simulink model "Ford_T3T6_ArchCnctnDigrm"  (R2016b)
settings: Solver=FixedStepDiscrete  StartTime=0.0  StopTime=10.0  RelTol=1e-3  EnableMultiTasking=on
libraries: canmsglib x15
(part 9 of 15)

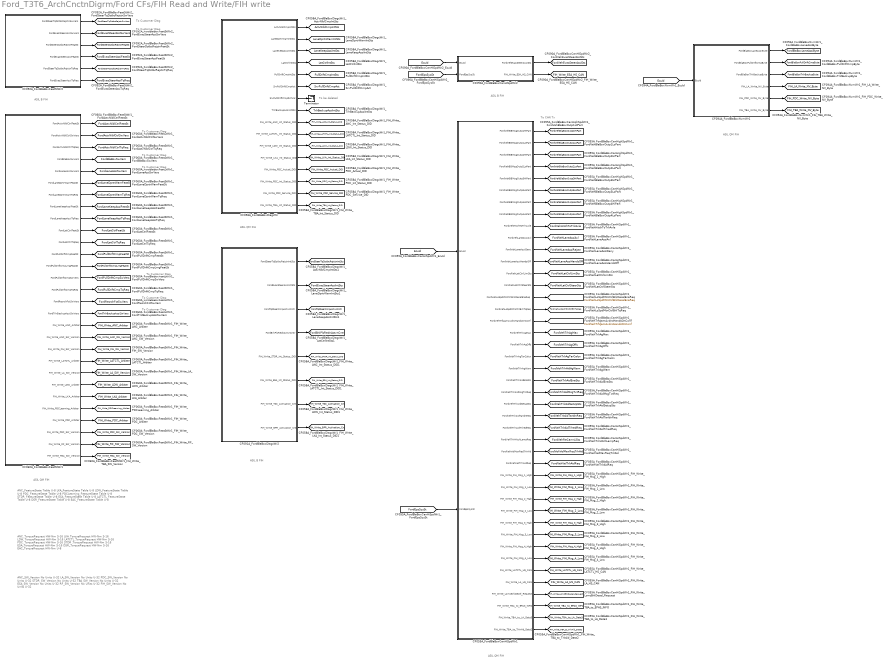
== system Ford_T3T6_ArchCnctnDigrm/Ford CFs/FIH Read and Write/FIH write ==
  note: ASIL QM FIH
  note: ASIL QM FIH
  note: ASIL B FIH
  note: ASIL B FIH
  note: ASIL QM FIH
  note: ASIL QM FIH
  note: ASIL B FIH
  note: To Customer Diag
  note: To be deleted
  note: To CAN Tx
  note: ANC_SW_Version
      | No Units
      | U-32
      |
      | LA_SW_Version
      | No Units
      | U-32
      |
      | PDC_SW_Version
      | No Units
      | U-32
      |
      | STDR_SW_Version
      | No Units
      | U-32
      |
      | TBA_SW_Version
      | No Units
      | U-32
      |
      | ESA_SW_Version
      | No Units
      | U-32
      |
      | RF_SW_Version
      | No Units
      | U-32
      |
      | FIH_SW_Version
      | No Units
      | U-32
  note: ANC_TorqueRequest
      | HW-Nm
      | S-16
      |
      | LKA_TorqueRequest
      | HW-Nm
      | S-16
      |
      | LDW_TorqueRequest
      | HW-Nm
      | S-16
      |
      | LATCTL_TorqueRequest
      | HW-Nm
      | S-16
      |
      | PDC_TorqueRequest
      | HW-Nm
      | S-16
      |
      | STDR_TorqueRequest
      | HW-Nm
      | S-16
      |
      | ESA_TorqueRequest
      | HW-Nm
      | S-16
      |
      | DSR_TorqueRequest
      | HW-Nm
      | S-16
      |
      | EAC_TorqueRequest
      | HW-Nm
      | U-8
  note: ANC_FeatureState
      | Table
      | U-8
      |
      | LKA_FeatureState
      | Table
      | U-8
      |
      | LDW_FeatureState
      | Table
      | U-8
      |
      | PDC_FeatureState
      | Table
      | U-8
      |
      | PDCLearning_FeatureState
      | Table
      | U-8
      |
      | STDR_FeatureState
      | Table
      | U-8
      |
      | ESA_FeatureState
      | Table
      | U-8
      |
      | LATCTL_FeatureState
      | Table
      | U-8
      |
      | DSR_FeatureState
      | Table
      | U-8
      |
      | EAC_FeatureState
      | Table
      | U-8
  note: To Customer Diag
  note: To Customer Diag
  note: To Customer Diag
  note: To Customer Diag
  note: To Customer Diag
  note: To Customer Diag
  note: To Customer Diag
  CF055A_FordBlaBoxCanHiSpdWr1 : Subsystem  Tag=1.0.X  Description=This function passes signals from Ford In House (FIH) features to the CAN bus. This function has no inputs as it is passing through data to the CAN bus from FIH.
      settings: AttributesFormatString=Version: %<Tag>
  CF058A_FordBlaBoxDiagcWr : Subsystem  Tag=1.0.X  Description=The Ford Black Box Diagnostic Write 1 function passes diagnosticinformation from Ford In House (FIH) features to the EPS.
      settings: AttributesFormatString=Version: %<Tag>
  CF060A_FordBlaBoxFeatStWr1 : Subsystem  Tag=1.0.X  Description=The Ford Black Box Feature State Write 1 function allows the Ford In-House (FIH) software,to write information to memory via a specified function call.
      settings: AttributesFormatString=Version: %<Tag>
  CF090A_FordBlaBoxCanHiSpdWr2 : Subsystem  Tag=1.0.X  Description=This function passes signals from Ford In House (FIH) features to the CAN bus. This function has no inputs as it is passing through data to the CAN bus from FIH.
      settings: AttributesFormatString=Version: %<Tag>
  CF091A_FordBlaBoxDiagcWr2 : Subsystem  Tag=1.0.X  Description=The Ford Black Box Diagnostic Write 2 function passes diagnosticinformation from Ford In House (FIH) features to the EPS.
      settings: AttributesFormatString=Version: %<Tag>
  CF092A_FordBlaBoxFeatStWr2 : Subsystem  Tag=1.0.X  Description=The Ford Black Box Feature State Write 2 function allows the Ford In-House (FIH) software, to write information to memory via a specified function call.
      settings: AttributesFormatString=Version: %<Tag>
  CF094A_FordBlaBoxNvmWr1 : Subsystem  Tag=1.0.X  Description=This function allows Ford In House features to read from and write to their specific NVM locations.
      settings: AttributesFormatString=Version: %<Tag>
  Terminator : Terminator
  tag scope: ActvNiblCmpIntSts=global, FIH_LA_Write_NV_Byte=global, FIH_PDC_Write_NV_Byte=global, FIH_TBA_Write_NV_Byte=global, FIH_Write_ANC_Arbiter=global, FIH_Write_ANC_Int_Status_DID=global, FIH_Write_ANC_SW_Version=global, FIH_Write_BPR_Activation_Cnt=global, FIH_Write_ESA_HS_CAN=global, FIH_Write_ESA_Int_Status_DID=global, FIH_Write_FIH_Msg_1_High=global, FIH_Write_FIH_Msg_1_Low=global, FIH_Write_FIH_Msg_2_High=global, FIH_Write_FIH_Msg_2_Low=global, FIH_Write_FIH_Msg_3_High=global, FIH_Write_FIH_Msg_3_Low=global, FIH_Write_FIH_Msg_4_High=global, FIH_Write_FIH_Msg_4_Low=global, FIH_Write_FIH_SW_Version=global, FIH_Write_LATCTL_Arbiter=global, FIH_Write_LATCTL_HS_CAN=global, FIH_Write_LATCTL_Int_Status_DID=global, FIH_Write_LA_HS_CAN=global, FIH_Write_LA_SW_Version=global, FIH_Write_LDW_Arbiter=global, FIH_Write_LDW_Int_Status_DID=global, FIH_Write_LKA_Arbiter=global, FIH_Write_LKA_Int_Status_DID=global, FIH_Write_LsmcBrkDecel_Request=global, FIH_Write_PDCLearning_Arbiter=global, FIH_Write_PDC_Actual_DID=global, FIH_Write_PDC_Arbiter=global, FIH_Write_PDC_Int_Status_DID=global, FIH_Write_PDC_SW_Version=global, FIH_Write_PDC_Service_DID=global, FIH_Write_RF_SW_Version=global, FIH_Write_STDR_Int_Status_DID=global, FIH_Write_TBA_Int_Status_DID=global, FIH_Write_TBA_SW_Version=global, FIH_Write_TBA_to_EPAS_INFO=global, FIH_Write_TBA_to_LA_Data3=global, FIH_Write_TBA_to_TrlrAid_Data2=global, FIH_Write_TSC_Activation_Cnt=global, FordActvNiblCtrlFeatSt=global, FordActvNiblCtrlSwVers=global, FordActvNiblCtrlTqReq=global, FordBlaBoxLaneAssiByte=global, FordBlaBoxPullDriftCmpByte=global, FordBlaBoxSwVers=global, FordBlaBoxTrlrBackupByte=global, FordBrkPlsRednActvnCntr=global, FordEvasSteerAssiFeatSt=global, FordEvasSteerAssiIntSts=global, FordEvasSteerAssiSwVers=global, FordEvasSteerAssiTqReq=global, FordLaneAssiSwVers=global, FordLaneDprtrWarnFeatSt=global, FordLaneDprtrWarnTqReq=global, FordLaneKeepAssiFeatSt=global, FordLaneKeepAssiTqReq=global, FordLatCtrlFeatSt=global, FordLatCtrlTqReq=global, FordPullDriftCmpFeatSt=global, FordPullDriftCmpLrngFeatSt=global, FordPullDriftCmpSwVers=global, FordPullDriftCmpTqReq=global, FordResrchFctSwVers=global, FordSteerDstbcRejctnFeatSt=global, FordSteerTqDstbcRejctnIntSts=global, FordSteerTqDstbcRejctnSwVers=global, FordSteerTqDstbcRejctnTqReq=global, FordTqSteerCmpActvnCntr=global, FordTrlrBackupAssiSwVers=global, FordVehBlaBoxOutp1HiPart=global, FordVehBlaBoxOutp1LoPart=global, FordVehBlaBoxOutp2HiPart=global, FordVehBlaBoxOutp2LoPart=global, FordVehBlaBoxOutp3HiPart=global, FordVehBlaBoxOutp3LoPart=global, FordVehBlaBoxOutp4HiPart=global, FordVehBlaBoxOutp4LoPart=global, FordVehEvasSteerAssiSts=global, FordVehHitchToTrlrAxle=global, FordVehLaneAssiAvl=global, FordVehLaneAssiHandsOff=global, FordVehLaneAssiRejctn=global, FordVehLatCtrlLimSts=global, FordVehLatCtrlSteerSts=global, FordVehLoSpdMtnCtrlBrkDecelEnaReq=global, FordVehLoSpdMtnCtrlBrkTqReq=global, FordVehReCamrLiSts=global, FordVehTrfcJamAvdncHandsOnConf=global, FordVehTrlrAgMax=global, FordVehTrlrAgOffs=global, FordVehTrlrAgTarCalcn=global, FordVehTrlrAidAgWarn=global, FordVehTrlrAidEnaSts=global, FordVehTrlrAidMsgTxtReq=global, FordVehTrlrAidSetUpSts=global, FordVehTrlrAidTarIdnReq=global, FordVehTrlrAidTrlredReq=global, FordVehVelMaxReqTrlrAid=global, FordVehVelTrlrAidReq=global, LaneDprtrWarnIntSts=global, LaneKeepAssiIntSts=global, LatCtrlIntSts=global, PullDriftCmpIntSts=global, SrvPullDriftCmpAct=global, TrlrBackupAssiIntSts=global
  wires:
  CF060A_FordBlaBoxFeatStWr1/1(FordActvNiblCtrlFeatSt) -> [FordActvNiblCtrlFeatSt]
  CF060A_FordBlaBoxFeatStWr1/2(FordActvNiblCtrlSwVers) -> [FordActvNiblCtrlSwVers]
  CF060A_FordBlaBoxFeatStWr1/3(FordActvNiblCtrlTqReq) -> [FordActvNiblCtrlTqReq]
  CF060A_FordBlaBoxFeatStWr1/4(FordBlaBoxSwVers) -> [FordBlaBoxSwVers]
  CF060A_FordBlaBoxFeatStWr1/5(FordLaneAssiSwVers) -> [FordLaneAssiSwVers]
  CF060A_FordBlaBoxFeatStWr1/6(FordLaneDprtrWarnFeatSt) -> [FordLaneDprtrWarnFeatSt]
  CF060A_FordBlaBoxFeatStWr1/7(FordLaneDprtrWarnTqReq) -> [FordLaneDprtrWarnTqReq]
  CF060A_FordBlaBoxFeatStWr1/8(FordLaneKeepAssiFeatSt) -> [FordLaneKeepAssiFeatSt]
  CF060A_FordBlaBoxFeatStWr1/9(FordLaneKeepAssiTqReq) -> [FordLaneKeepAssiTqReq]
  CF060A_FordBlaBoxFeatStWr1/10(FordLatCtrlFeatSt) -> [FordLatCtrlFeatSt]
  CF060A_FordBlaBoxFeatStWr1/11(FordLatCtrlTqReq) -> [FordLatCtrlTqReq]
  CF060A_FordBlaBoxFeatStWr1/12(FordPullDriftCmpFeatSt) -> [FordPullDriftCmpFeatSt]
  CF060A_FordBlaBoxFeatStWr1/13(FordPullDriftCmpLrngFeatSt) -> [FordPullDriftCmpLrngFeatSt]
  CF060A_FordBlaBoxFeatStWr1/14(FordPullDriftCmpSwVers) -> [FordPullDriftCmpSwVers]
  CF060A_FordBlaBoxFeatStWr1/15(FordPullDriftCmpTqReq) -> [FordPullDriftCmpTqReq]
  CF060A_FordBlaBoxFeatStWr1/16(FordResrchFctSwVers) -> [FordResrchFctSwVers]
  CF060A_FordBlaBoxFeatStWr1/17(FordTrlrBackupAssiSwVers) -> [FordTrlrBackupAssiSwVers]
  CF060A_FordBlaBoxFeatStWr1/18(FIH_Write_ANC_Arbiter) -> [FIH_Write_ANC_Arbiter]
  CF060A_FordBlaBoxFeatStWr1/19(FIH_Write_ANC_SW_Version) -> [FIH_Write_ANC_SW_Version]
  CF060A_FordBlaBoxFeatStWr1/20(FIH_Write_FIH_SW_Version) -> [FIH_Write_FIH_SW_Version]
  CF060A_FordBlaBoxFeatStWr1/21(FIH_Write_LATCTL_Arbiter) -> [FIH_Write_LATCTL_Arbiter]
  CF060A_FordBlaBoxFeatStWr1/22(FIH_Write_LA_SW_Version) -> [FIH_Write_LA_SW_Version]
  CF060A_FordBlaBoxFeatStWr1/23(FIH_Write_LDW_Arbiter) -> [FIH_Write_LDW_Arbiter]
  CF060A_FordBlaBoxFeatStWr1/24(FIH_Write_LKA_Arbiter) -> [FIH_Write_LKA_Arbiter]
  CF060A_FordBlaBoxFeatStWr1/25(FIH_Write_PDCLearning_Arbiter) -> [FIH_Write_PDCLearning_Arbiter]
  CF060A_FordBlaBoxFeatStWr1/26(FIH_Write_PDC_Arbiter) -> [FIH_Write_PDC_Arbiter]
  CF060A_FordBlaBoxFeatStWr1/27(FIH_Write_PDC_SW_Version) -> [FIH_Write_PDC_SW_Version]
  CF060A_FordBlaBoxFeatStWr1/28(FIH_Write_RF_SW_Version) -> [FIH_Write_RF_SW_Version]
  CF060A_FordBlaBoxFeatStWr1/29(FIH_Write_TBA_SW_Version) -> [FIH_Write_TBA_SW_Version]
  CF058A_FordBlaBoxDiagcWr/1(ActvNiblCmpIntSts) -> [ActvNiblCmpIntSts]
  CF058A_FordBlaBoxDiagcWr/2(LaneDprtrWarnIntSts) -> [LaneDprtrWarnIntSts]
  CF058A_FordBlaBoxDiagcWr/3(LaneKeepAssiIntSts) -> [LaneKeepAssiIntSts]
  CF058A_FordBlaBoxDiagcWr/4(LatCtrlIntSts) -> [LatCtrlIntSts]
  CF058A_FordBlaBoxDiagcWr/5(PullDriftCmpIntSts) -> [PullDriftCmpIntSts]
  CF058A_FordBlaBoxDiagcWr/6(SrvPullDriftCmpAct) -> [SrvPullDriftCmpAct]
  CF058A_FordBlaBoxDiagcWr/7(SrvPullDriftCmpRstVal) -> Terminator/1
  CF058A_FordBlaBoxDiagcWr/8(TrlrBackupAssiIntSts) -> [TrlrBackupAssiIntSts]
  CF058A_FordBlaBoxDiagcWr/9(FIH_Write_ANC_Int_Status_DID) -> [FIH_Write_ANC_Int_Status_DID]
  CF058A_FordBlaBoxDiagcWr/10(FIH_Write_LATCTL_Int_Status_DID) -> [FIH_Write_LATCTL_Int_Status_DID]
  CF058A_FordBlaBoxDiagcWr/11(FIH_Write_LDW_Int_Status_DID) -> [FIH_Write_LDW_Int_Status_DID]
  CF058A_FordBlaBoxDiagcWr/12(FIH_Write_LKA_Int_Status_DID) -> [FIH_Write_LKA_Int_Status_DID]
  CF058A_FordBlaBoxDiagcWr/13(FIH_Write_PDC_Actual_DID) -> [FIH_Write_PDC_Actual_DID]
  CF058A_FordBlaBoxDiagcWr/14(FIH_Write_PDC_Int_Status_DID) -> [FIH_Write_PDC_Int_Status_DID]
  CF058A_FordBlaBoxDiagcWr/15(FIH_Write_PDC_Service_DID) -> [FIH_Write_PDC_Service_DID]
  CF058A_FordBlaBoxDiagcWr/16(FIH_Write_TBA_Int_Status_DID) -> [FIH_Write_TBA_Int_Status_DID]
  [EcuId] -> CF090A_FordBlaBoxCanHiSpdWr2/1(EcuId)
  [FordEpsSysSt] -> CF090A_FordBlaBoxCanHiSpdWr2/2(FordEpsSysSt)
  CF090A_FordBlaBoxCanHiSpdWr2/1(FordVehEvasSteerAssiSts) -> [FordVehEvasSteerAssiSts]
  CF090A_FordBlaBoxCanHiSpdWr2/2(FIH_Write_ESA_HS_CAN) -> [FIH_Write_ESA_HS_CAN]
  [EcuId] -> CF094A_FordBlaBoxNvmWr1/1(EcuId)
  CF094A_FordBlaBoxNvmWr1/1(FordBlaBoxLaneAssiByte) -> [FordBlaBoxLaneAssiByte]
  CF094A_FordBlaBoxNvmWr1/2(FordBlaBoxPullDriftCmpByte) -> [FordBlaBoxPullDriftCmpByte]
  CF094A_FordBlaBoxNvmWr1/3(FordBlaBoxTrlrBackupByte) -> [FordBlaBoxTrlrBackupByte]
  CF094A_FordBlaBoxNvmWr1/4(FIH_LA_Write_NV_Byte) -> [FIH_LA_Write_NV_Byte]
  CF094A_FordBlaBoxNvmWr1/5(FIH_PDC_Write_NV_Byte) -> [FIH_PDC_Write_NV_Byte]
  CF094A_FordBlaBoxNvmWr1/6(FIH_TBA_Write_NV_Byte) -> [FIH_TBA_Write_NV_Byte]
  CF092A_FordBlaBoxFeatStWr2/1(FordSteerTqDstbcRejctnSwVers) -> [FordSteerTqDstbcRejctnSwVers]
  CF092A_FordBlaBoxFeatStWr2/2(FordEvasSteerAssiSwVers) -> [FordEvasSteerAssiSwVers]
  CF092A_FordBlaBoxFeatStWr2/3(FordSteerDstbcRejctnFeatSt) -> [FordSteerDstbcRejctnFeatSt]
  CF092A_FordBlaBoxFeatStWr2/4(FordEvasSteerAssiFeatSt) -> [FordEvasSteerAssiFeatSt]
  CF092A_FordBlaBoxFeatStWr2/5(FordSteerTqDstbcRejctnTqReq) -> [FordSteerTqDstbcRejctnTqReq]
  CF092A_FordBlaBoxFeatStWr2/6(FordEvasSteerAssiTqReq) -> [FordEvasSteerAssiTqReq]
  [EcuId] -> CF055A_FordBlaBoxCanHiSpdWr1/1(EcuId)
  [FordEpsSysSt] -> CF055A_FordBlaBoxCanHiSpdWr1/2(FordEpsSysSt)
  CF055A_FordBlaBoxCanHiSpdWr1/1(FordVehBBMsgOutp1HiPart) -> [FordVehBlaBoxOutp1HiPart]
  CF055A_FordBlaBoxCanHiSpdWr1/2(FordVehBBMsgOutp1LoPart) -> [FordVehBlaBoxOutp1LoPart]
  CF055A_FordBlaBoxCanHiSpdWr1/3(FordVehBBMsgOutp2HiPart) -> [FordVehBlaBoxOutp2HiPart]
  CF055A_FordBlaBoxCanHiSpdWr1/4(FordVehBBMsgOutp2LoPart) -> [FordVehBlaBoxOutp2LoPart]
  CF055A_FordBlaBoxCanHiSpdWr1/5(FordVehBBMsgOutp3HiPart) -> [FordVehBlaBoxOutp3HiPart]
  CF055A_FordBlaBoxCanHiSpdWr1/6(FordVehBBMsgOutp3LoPart) -> [FordVehBlaBoxOutp3LoPart]
  CF055A_FordBlaBoxCanHiSpdWr1/7(FordVehBBMsgOutp4HiPart) -> [FordVehBlaBoxOutp4HiPart]
  CF055A_FordBlaBoxCanHiSpdWr1/8(FordVehBBMsgOutp4LoPart) -> [FordVehBlaBoxOutp4LoPart]
  CF055A_FordBlaBoxCanHiSpdWr1/9(FordVehHitchToTrlrAxle) -> [FordVehHitchToTrlrAxle]
  CF055A_FordBlaBoxCanHiSpdWr1/10(FordVehLaneAssiAvl) -> [FordVehLaneAssiAvl]
  CF055A_FordBlaBoxCanHiSpdWr1/11(FordVehLaneAssiDeny) -> [FordVehLaneAssiRejctn]
  CF055A_FordBlaBoxCanHiSpdWr1/12(FordVehLaneAssiHandsOff) -> [FordVehLaneAssiHandsOff]
  CF055A_FordBlaBoxCanHiSpdWr1/13(FordVehLatCtrlLimSts) -> [FordVehLatCtrlLimSts]
  CF055A_FordBlaBoxCanHiSpdWr1/14(FordVehLatCtrlSteerSts) -> [FordVehLatCtrlSteerSts]
  CF055A_FordBlaBoxCanHiSpdWr1/15(FordVehLoSpdMtnCtrlBrkDecelEnaReq) -> [FordVehLoSpdMtnCtrlBrkDecelEnaReq]
  CF055A_FordBlaBoxCanHiSpdWr1/16(FordVehLoSpdMtnCtrlBrkTqReq) -> [FordVehLoSpdMtnCtrlBrkTqReq]
  CF055A_FordBlaBoxCanHiSpdWr1/17(FordVehTrfcJamAvdncHandsOnConf) -> [FordVehTrfcJamAvdncHandsOnConf]
  CF055A_FordBlaBoxCanHiSpdWr1/18(FordVehTrlrAgMax) -> [FordVehTrlrAgMax]
  CF055A_FordBlaBoxCanHiSpdWr1/19(FordVehTrlrAgOffs) -> [FordVehTrlrAgOffs]
  CF055A_FordBlaBoxCanHiSpdWr1/20(FordVehTrlrAgTarCalcn) -> [FordVehTrlrAgTarCalcn]
  CF055A_FordBlaBoxCanHiSpdWr1/21(FordVehTrlrAgWarn) -> [FordVehTrlrAidAgWarn]
  CF055A_FordBlaBoxCanHiSpdWr1/22(FordVehTrlrAidEnaSts) -> [FordVehTrlrAidEnaSts]
  CF055A_FordBlaBoxCanHiSpdWr1/23(FordVehTrlrAidMsgTxtReq) -> [FordVehTrlrAidMsgTxtReq]
  CF055A_FordBlaBoxCanHiSpdWr1/24(FordVehTrlrAidSetupSts) -> [FordVehTrlrAidSetUpSts]
  CF055A_FordBlaBoxCanHiSpdWr1/25(FordVehTrlrAidTarIdnReq) -> [FordVehTrlrAidTarIdnReq]
  CF055A_FordBlaBoxCanHiSpdWr1/26(FordVehTrlrAidTrlredReq) -> [FordVehTrlrAidTrlredReq]
  CF055A_FordBlaBoxCanHiSpdWr1/27(FordVehTrlrHitchLampReq) -> [FordVehReCamrLiSts]
  CF055A_FordBlaBoxCanHiSpdWr1/28(FordVehVelMaxReqTrlrAid) -> [FordVehVelMaxReqTrlrAid]
  CF055A_FordBlaBoxCanHiSpdWr1/29(FordVehVelTrlrAidReq) -> [FordVehVelTrlrAidReq]
  CF055A_FordBlaBoxCanHiSpdWr1/30(FIH_Write_FIH_Msg_1_High) -> [FIH_Write_FIH_Msg_1_High]
  CF055A_FordBlaBoxCanHiSpdWr1/31(FIH_Write_FIH_Msg_1_Low) -> [FIH_Write_FIH_Msg_1_Low]
  CF055A_FordBlaBoxCanHiSpdWr1/32(FIH_Write_FIH_Msg_2_High) -> [FIH_Write_FIH_Msg_2_High]
  CF055A_FordBlaBoxCanHiSpdWr1/33(FIH_Write_FIH_Msg_2_Low) -> [FIH_Write_FIH_Msg_2_Low]
  CF055A_FordBlaBoxCanHiSpdWr1/34(FIH_Write_FIH_Msg_3_High) -> [FIH_Write_FIH_Msg_3_High]
  CF055A_FordBlaBoxCanHiSpdWr1/35(FIH_Write_FIH_Msg_3_Low) -> [FIH_Write_FIH_Msg_3_Low]
  CF055A_FordBlaBoxCanHiSpdWr1/36(FIH_Write_FIH_Msg_4_High) -> [FIH_Write_FIH_Msg_4_High]
  CF055A_FordBlaBoxCanHiSpdWr1/37(FIH_Write_FIH_Msg_4_Low) -> [FIH_Write_FIH_Msg_4_Low]
  CF055A_FordBlaBoxCanHiSpdWr1/38(FIH_Write_LATCTL_HS_CAN) -> [FIH_Write_LATCTL_HS_CAN]
  CF055A_FordBlaBoxCanHiSpdWr1/39(FIH_Write_LA_HS_CAN) -> [FIH_Write_LA_HS_CAN]
  CF055A_FordBlaBoxCanHiSpdWr1/40(FIH_Write_LsmcBrkDecel_Request) -> [FIH_Write_LsmcBrkDecel_Request]
  CF055A_FordBlaBoxCanHiSpdWr1/41(FIH_Write_TBA_to_EPAS_INFO) -> [FIH_Write_TBA_to_EPAS_INFO]
  CF055A_FordBlaBoxCanHiSpdWr1/42(FIH_Write_TBA_to_LA_Data3) -> [FIH_Write_TBA_to_LA_Data3]
  CF055A_FordBlaBoxCanHiSpdWr1/43(FIH_Write_TBA_to_TrlrAid_Data2) -> [FIH_Write_TBA_to_TrlrAid_Data2]
  CF091A_FordBlaBoxDiagcWr2/1(FordSteerTqDstbcRejctnIntSts) -> [FordSteerTqDstbcRejctnIntSts]
  CF091A_FordBlaBoxDiagcWr2/2(FordEvasSteerAssiIntSts) -> [FordEvasSteerAssiIntSts]
  CF091A_FordBlaBoxDiagcWr2/3(FordTqSteerCmpActvnCntr) -> [FordTqSteerCmpActvnCntr]
  CF091A_FordBlaBoxDiagcWr2/4(FordBrkPlsRednActvnCntr) -> [FordBrkPlsRednActvnCntr]
  CF091A_FordBlaBoxDiagcWr2/5(FIH_Write_STDR_Int_Status_DID) -> [FIH_Write_STDR_Int_Status_DID]
  CF091A_FordBlaBoxDiagcWr2/6(FIH_Write_ESA_Int_Status_DID) -> [FIH_Write_ESA_Int_Status_DID]
  CF091A_FordBlaBoxDiagcWr2/7(FIH_Write_TSC_Activation_Cnt) -> [FIH_Write_TSC_Activation_Cnt]
  CF091A_FordBlaBoxDiagcWr2/8(FIH_Write_BPR_Activation_Cnt) -> [FIH_Write_BPR_Activation_Cnt]

== system Ford_T3T6_ArchCnctnDigrm/Ford CFs/Internal CF/CF046A_FordVltgIf ==
  BattRtnCurr : Inport
  BattRtnCurrImc : Inport  Port=2
  BattVltg : Inport  Port=3
  FordActvParkAssiEnad : Inport  Port=4
  FordEpsSysSt : Inport  Port=5
  FordEvasSteerAssiEnad : Inport  Port=6
  FordLaneCentrAssiEnad : Inport  Port=7
  FordLaneDprtrWarnEnad : Inport  Port=8
  FordLaneKeepAssiEnad : Inport  Port=9
  FordMaxAsscTq : Inport  Port=10
  FordSysSt : Inport  Port=11
  FordTrfcJamAssiEnad : Inport  Port=12
  FordTrlrBackupAssiEnad : Inport  Port=13
  FordVehElecPwrStrtStopSts : Inport  Port=14
  FordVehElecPwrSts : Inport  Port=15
  FordVehIgnStsQly : Inport  Port=16
  FordVehPwrpkTqSts : Inport  Port=17
  FordVehSpd : Inport  Port=18
  FordVehSpdVld : Inport  Port=19
  GetRefTmr100MicroSec32bit : Inport  Port=20
  GetTiSpan100MicroSec32bit : Inport  Port=21
  SetNtcSts : Inport  Port=22
  FordEpsCurr : Outport
  FordEpsVltg : Outport  Port=2
  FordFeatThdSts : Outport  Port=3
  FordInhbBattVltgDiagc : Outport  Port=4
  FordMaxBattCurr : Outport  Port=5
  FordMinBattVltg : Outport  Port=6
  FordVltgOperRamp : Outport  Port=7
  FordVltgOperScar : Outport  Port=8
  FordVltgOperSt : Outport  Port=9

== system Ford_T3T6_ArchCnctnDigrm/Ford CFs/Internal CF/CF047A_FordStrtStop ==
  CmpdSteerPinionAg : Inport
  CmpdSteerPinionAgQlyFac : Inport  Port=2
  EcuId : Inport  Port=3
  FildVehSpd : Inport  Port=4
  FordBoostCrvInpTq : Inport  Port=5
  FordCanDtcInhb : Inport  Port=6
  FordEpsSysSt : Inport  Port=7
  FordVehElecPwrStrtStopSts : Inport  Port=8
  SteerPinionAgVel : Inport  Port=9
  SteerPinionAgVelVld : Inport  Port=10
  StrtStopDIDSt : Inport  Port=11
  GetRefTmr100MicroSec32bit : Inport  Port=12
  GetSigImcData_logl : Inport  Port=13
  GetSigImcData_u08 : Inport  Port=14
  GetTiSpan100MicroSec32bit : Inport  Port=15
  FordIntPwrReqSt : Outport
  FordIntStrtStopSt : Outport  Port=2
  FordPwrReqSt : Outport  Port=3
  SysOperMotTqCmdSca : Outport  Port=4
  SysOperRampRate : Outport  Port=5

== system Ford_T3T6_ArchCnctnDigrm/Ford CFs/Internal CF/CF048A_DrvrSteerRcmdn ==
  DSRVld : Inport
  DSR_ArbiterCmd : Inport  Port=2
  DSR_Enad : Inport  Port=3
  DrvSte_D_Stat : Inport  Port=4
  DrvSte_Tq_Rq : Inport  Port=5
  EcuId : Inport  Port=6
  RvsGearVld : Inport  Port=7
  VehSpdVld : Inport  Port=8
  GetImcSigData_f32 : Inport  Port=9
  GetImcSigData_logl : Inport  Port=10
  GetImcSigData_u08 : Inport  Port=11
  DSR_FeatSt_PostImc : Outport
  DSR_FeatSt_PreImc : Outport  Port=2
  DSR_TqReq_PostImc : Outport  Port=3
  DSR_TqReq_PreImc : Outport  Port=4
  DrvSteAct_B_Stat_PostImc : Outport  Port=5
  DrvSteAct_B_Stat_PreImc : Outport  Port=6
  DrvSte_Tq_Act : Outport  Port=7

== system Ford_T3T6_ArchCnctnDigrm/Ford CFs/Internal CF/CF050A_FordCanDtcInhb ==
  EcuId : Inport
  FordBattVltgEstimn : Inport  Port=2
  FordEpsSysSt : Inport  Port=3
  FordVehElecPwrSts : Inport  Port=4
  FordVehIgnStsQly : Inport  Port=5
  FordVehLifeCycModQly : Inport  Port=6
  FordVehPwrpkTqSts : Inport  Port=7
  GetRefTmr100MicroSec32bit : Inport  Port=8
  GetSigImcData_logl : Inport  Port=9
  GetSigImcData_u08 : Inport  Port=10
  GetTiSpan100MicroSec32bit : Inport  Port=11
  IoHwAb_GetGpioMcuEna : Inport  Port=12
  OdomMstVal : Inport  Port=13
  FordCanDtcInhb : Outport
  FordEpsLifeCycMod : Outport  Port=2

== system Ford_T3T6_ArchCnctnDigrm/Ford CFs/Internal CF/CF052A_FordSysSt ==
  IoHwAb_GetGpioMcuEna : Inport
  LoaSt : Inport  Port=2
  SysSt : Inport  Port=3
  FordVehPwrpkTqSts : Inport  Port=4
  FordVehSpd : Inport  Port=5
  FordVehSpdVld : Inport  Port=6
  FordVltgOperSt : Inport  Port=7
  GetNtcQlfrSts : Inport  Port=8
  FordEpsFailr : Outport
  FordEpsSysSt : Outport  Port=2
  FordPwrSplyEnaReq : Outport  Port=3
  FordSteerModlSts : Outport  Port=4
  FordEpsEna : Outport  Port=5
  FordSysStReqEna : Outport  Port=6

== system Ford_T3T6_ArchCnctnDigrm/Ford CFs/Internal CF/CF063A_DrvgSteerSel ==
  ActvRtIdx : Inport
  BoostCrvInpTq : Inport  Port=2
  EcuId : Inport  Port=3
  EpsSysSt : Inport  Port=4
  FltMtgtn : Inport  Port=5
  LoaSt : Inport  Port=6
  SelvDrvgModChassis2Req : Inport  Port=7
  SelvDrvgModChassisVld : Inport  Port=8
  SelvDrvgModEnad : Inport  Port=9
  VehSpd : Inport  Port=10
  VehSpdVld : Inport  Port=11
  GetRefTmr100MicroSec32bit : Inport  Port=12
  GetSigImcData_u08 : Inport  Port=13
  GetTiSpan100MicroSec32bit : Inport  Port=14
  RtCalChgReqSts : Outport
  SelvDrvgModSteerModReq : Outport  Port=2
  SelvDrvgModSteerSts : Outport  Port=3
  XcpCalChgReqSts : Outport  Port=4
  RtReqSrv : Outport  Port=5
  XcpReqSrv : Outport  Port=6

== system Ford_T3T6_ArchCnctnDigrm/Ford CFs/Internal CF/CF065A_FordCmdArbn ==
  EcuId : Inport
  FordActvNiblCtrlFeatSt : Inport  Port=2
  FordDrvrSteerRcmdnFeatSt : Inport  Port=3
  FordEvasSteerAssiFeatSt : Inport  Port=4
  FordExtAgCtrlFeatSt : Inport  Port=5
  FordLaneDprtrWarnFeatSt : Inport  Port=6
  FordLaneKeepAssiFeatSt : Inport  Port=7
  FordLatCtrlFeatSt : Inport  Port=8
  FordMaxAssiTq : Inport  Port=9
  FordPullDriftCmpFeatSt : Inport  Port=10
  FordPullDriftCmpLrngFeatSt : Inport  Port=11
  FordSpare1FeatSt : Inport  Port=12
  FordSpare2FeatSt : Inport  Port=13
  FordSpare3FeatSt : Inport  Port=14
  FordSteerDstbcRejctnFeatSt : Inport  Port=15
  FordSteerModlSts : Inport  Port=16
  GetSigImcData_u08 : Inport  Port=17
  FordActvNiblCtrlArbnCmd : Outport
  FordDrvrSteerRcmdnArbnCmd : Outport  Port=2
  FordEvasSteerAssiArbnCmd : Outport  Port=3
  FordExtAgCtrlArbnCmd : Outport  Port=4
  FordLaneDprtrWarnArbnCmd : Outport  Port=5
  FordLaneKeepAssiArbnCmd : Outport  Port=6
  FordLatCtrlArbnCmd : Outport  Port=7
  FordPullDriftCmpArbnCmd : Outport  Port=8
  FordPullDriftCmpLrngArbnCmd : Outport  Port=9
  FordSpare1ArbnCmd : Outport  Port=10
  FordSpare2ArbnCmd : Outport  Port=11
  FordSpare3ArbnCmd : Outport  Port=12
  FordSteerDstbcRejctnArbnCmd : Outport  Port=13

== system Ford_T3T6_ArchCnctnDigrm/Ford CFs/Internal CF/CF066A_FordMotTqCmdOvrlLimr ==
  EcuId : Inport
  FildHwTq : Inport  Port=2
  FildVehSpd : Inport  Port=3
  FordActvNiblCtrlArbnCmd : Inport  Port=4
  FordActvNiblCtrlFctCallSts : Inport  Port=5
  FordActvNiblCtrlTqReq : Inport  Port=6
  FordLaneDprtrWarnArbnCmd : Inport  Port=7
  FordLaneDprtrWarnFctCallSts : Inport  Port=8
  FordLaneDprtrWarnTqReq : Inport  Port=9
  FordLatCtrlArbnCmd : Inport  Port=10
  FordLatCtrlFctCallSts : Inport  Port=11
  FordLatCtrlTqReq : Inport  Port=12
  FordPullDriftCmpArbnCmd : Inport  Port=13
  FordPullDriftCmpFctCallSts : Inport  Port=14
  FordPullDriftCmpTqReq : Inport  Port=15
  FordSteerTqDstbcRejctnArbnCmd : Inport  Port=16
  FordSteerTqDstbcRejctnFctCallSts : Inport  Port=17
  FordSteerTqDstbcRejctnTqReq : Inport  Port=18
  HwVel : Inport  Port=19
  VehSpdVld : Inport  Port=20
  GetRefTmr100MicroSec32bit : Inport  Port=21
  GetSigImcData_f32 : Inport  Port=22
  GetSigImcData_logl : Inport  Port=23
  GetTiSpan100MicroSec32bit : Inport  Port=24
  SetNtcSts : Inport  Port=25
  FordMotTqOvrl : Outport

== system Ford_T3T6_ArchCnctnDigrm/Ford CFs/Internal CF/CF067A_FordHwTqCmdOvrlLimr ==
  EcuId : Inport
  FildVehSpd : Inport  Port=2
  FordDrvrSteerRcmdnArbnCmd : Inport  Port=3
  FordDrvrSteerRcmdnFctCallSts : Inport  Port=4
  FordDrvrSteerRcmdnTqReq : Inport  Port=5
  FordEvasSteerAssiArbnCmd : Inport  Port=6
  FordEvasSteerAssiFctCallSts : Inport  Port=7
  FordEvasSteerAssiTqReq : Inport  Port=8
  FordLaneKeepAssiArbnCmd : Inport  Port=9
  FordLaneKeepAssiFctCallSts : Inport  Port=10
  FordLaneKeepAssiTqReq : Inport  Port=11
  VehSpdVld : Inport  Port=12
  GetSigImcData_f32 : Inport  Port=13
  GetSigImcData_logl : Inport  Port=14
  FordColTqOvrl : Outport

== system Ford_T3T6_ArchCnctnDigrm/Ford CFs/Internal CF/CF068A_FordExtAgCtrl ==
  ActvFrntSteerPrsnt : Inport
  AssiCmdBas : Inport  Port=2
  EcuId : Inport  Port=3
  ExtAgCtrlDiagcFlg : Inport  Port=4
  FildVehSpd : Inport  Port=5
  FordActvFrntSteerModlSteerWhlAgVldInt : Inport  Port=6
  FordActvParkAssiEnad : Inport  Port=7
  FordCmpdHwPosn : Inport  Port=8
  FordCmpdHwPosnQlyFac : Inport  Port=9
  FordEpsSysSt : Inport  Port=10
  FordRelHwPosn : Inport  Port=11
  FordTrlrBackupAssiEnad : Inport  Port=12
  FordVehActvFrntSteerModlSteerWhlAg : Inport  Port=13
  FordVehParkAidModlReqdAg : Inport  Port=14
  FordVehParkAidModlReqdSts : Inport  Port=15
  HwTq : Inport  Port=16
  HwVel : Inport  Port=17
  LeLeastDrvnVehSpd : Inport  Port=18
  PosnServoCmd : Inport  Port=19
  RiLeastDrvnVehSpd : Inport  Port=20
  VehSpdVld : Inport  Port=21
  GetRefTmr100MicroSec32bit : Inport  Port=22
  GetSigImcData_f32 : Inport  Port=23
  GetSigImcData_logl : Inport  Port=24
  GetTiSpan100MicroSec32bit : Inport  Port=25
  SetNtcSts : Inport  Port=26
  ExtAgCtrlStsInt : Outport
  ExtAgCtrlTqReq : Outport  Port=2
  PosnServoEna : Outport  Port=3
  PosnServoHwAg : Outport  Port=4
  SemiAutParlParkAgCtrlSts1 : Outport  Port=5
  SemiAutParlParkAgCtrlSts2 : Outport  Port=6
  SemiAutParlParkAgCtrlSts3 : Outport  Port=7
  SemiAutParlParkAgCtrlSts4 : Outport  Port=8
  SemiAutParlParkAgCtrlSts5 : Outport  Port=9
  SemiAutParlParkAgCtrlSts6 : Outport  Port=10
  FIH_Trailer_Backup_Assist_AngleRequest_Function : Outport  Port=11
  FIH_Trailer_Backup_Assist_External_Angle_ControlStatus_Function : Outport  Port=12

== system Ford_T3T6_ArchCnctnDigrm/Ford CFs/Internal CF/CF076A_FordHwTqCdng ==
  AssiCmd : Inport
  AssiCmdBas : Inport  Port=2
  FordVehSpd : Inport  Port=3
  HwTq : Inport  Port=4
  HwTqHysOvrl : Inport  Port=5
  HwTqOvrl : Inport  Port=6
  MotTqCmd : Inport  Port=7
  MotTqCmdPwrLimd : Inport  Port=8
  AvlMotTq : Inport  Port=9
  EcuId : Inport  Port=10
  GetNtcQlfrSts : Inport  Port=11
  GetRefTmr100MicroSec32bit : Inport  Port=12
  GetTiSpan100MicroSec32bit : Inport  Port=13
  FordAppldFinalMotTq : Outport
  FordAppldFinalMotTqVld : Outport  Port=2
  FordBoostCrvAssiTq : Outport  Port=3
  FordBoostCrvInpTq : Outport  Port=4
  FordFeatDircBCTq : Outport  Port=5
  FordInpTqRaw : Outport  Port=6
  FordInpTqRawVld : Outport  Port=7
  FordReqdFinalMotTq : Outport  Port=8
  FIH_Read_EPS_Direct_BC_Torque : Outport  Port=9
  FIH_Read_EPS_Inverse_BC_Torque : Outport  Port=10
  FordMaxAsscTq : Outport  Port=11

== system Ford_T3T6_ArchCnctnDigrm/Generate Steering Command/Openloop Steering Command/GenerateSteeringCommand ==
  note: SF063
  note: Taken Care by FIH
  note: CMS?
  note: ASIL D
  note: ASIL D
  note: Taken Care by FIH
  note: Taken Care by FIH
  note: SF063
  HwTqSwp : Inport
  EotAssiSca : Inport  Port=2
  EotActvCmd : Inport  Port=3
  EotDampgCmd : Inport  Port=4
  EotMotTqLim : Inport  Port=5
  StallMotTqLim : Inport  Port=6
  ThermMotTqLim : Inport  Port=7
  VehSpdMotTqLim : Inport  Port=8
  Assist : Subsystem
  Damping : Subsystem
  Ground{,1..6} (7 alike) : Ground
  Return : Subsystem
  SF004B_AssiSumLim : Subsystem  Tag=2.3.0  Description="This function sums torque commands from various functions and then limits the net command.  It serves as a focal point for safety crosschecks that may reside in Channel 2 memory."
      settings: AttributesFormatString=Version: %<Tag>
  SF020B_PosnTrakgServo : Subsystem  Tag=1.1.0  Description=This function provides the ability for the EPS system to track a position input command.
      settings: AttributesFormatString=Version: %<Tag>
  MotTqCmd : Outport
  MotTqCmdLimdPreStall : Outport  Port=2
  tag scope: MotTqCmd=global, MotTqCmdLimdPreStall=global, MotTqCmdLimrMin=global, MotTqCmdPreLim=global, PosnServoCmd=global, PosnServoIntgtrSt=global, SetManTqCmd=global, SysProtnRednFac=global
  wires:
  SF004B_AssiSumLim/1(MotTqCmd) -> MotTqCmd/1, [MotTqCmd]
  Assist/2(AssiCmdBas) -> Damping/1(AssiCmdBas)
  SF004B_AssiSumLim/2(MotTqCmdLimdPreStall) -> MotTqCmdLimdPreStall/1, [MotTqCmdLimdPreStall]
  HwTqSwp/1 -> Return/1(HwTqSwp), Damping/2(HwTqSwp), Assist/1(HwTqSwp)
  [HwAg] -> SF020B_PosnTrakgServo/1(HwAg)
  [HwTq] -> SF020B_PosnTrakgServo/2(HwTq)
  [MotVelCrf] -> SF020B_PosnTrakgServo/3(MotVelCrf)
  [PosnServoEna] -> SF020B_PosnTrakgServo/4(PosnServoEna)
  [PosnServoHwAg] -> SF020B_PosnTrakgServo/5(PosnServoHwAg)
  Ground6/1 -> SF020B_PosnTrakgServo/6(PosnServoHwVel)
  Ground5/1 -> SF020B_PosnTrakgServo/8(PosnTrakgArbnFltMtgtnEna)
  [VehSpd] -> SF020B_PosnTrakgServo/9(VehSpd)
  SF020B_PosnTrakgServo/2(PosnServoIntgtrSt) -> [PosnServoIntgtrSt]
  Ground4/1 -> SF020B_PosnTrakgServo/7(PosnServoIntgtrOffs)
  Assist/1(AssiCmd) -> SF004B_AssiSumLim/1(AssiCmd)
  Damping/1(DampgCmd) -> SF004B_AssiSumLim/2(DampgCmd)
  EotActvCmd/1 -> SF004B_AssiSumLim/3(EotActvCmd)
  EotAssiSca/1 -> SF004B_AssiSumLim/4(EotAssiSca)
  EotDampgCmd/1 -> SF004B_AssiSumLim/5(EotDampgCmd)
  EotMotTqLim/1 -> SF004B_AssiSumLim/6(EotMotTqLim)
  [HwTqLoaMtgtnEna] -> SF004B_AssiSumLim/7(HwTqLoaMtgtnEna)
  [MotTqCmdLimDi] -> SF004B_AssiSumLim/8(MotTqCmdLimDi)
  [MotVelMrf] -> SF004B_AssiSumLim/10(MotVelMrf)
  Ground/1 -> SF004B_AssiSumLim/12(PinionCentrLrnEna), SF004B_AssiSumLim/11(PinionCentrLrnCmd)
  Ground1/1 -> SF004B_AssiSumLim/13(PullCmpCmd)
  [PwrLimrRednFac] -> SF004B_AssiSumLim/14(PwrLimrRednFac)
  Return/1(RtnCmd) -> SF004B_AssiSumLim/15(RtnCmd)
  StallMotTqLim/1 -> SF004B_AssiSumLim/16(StallMotTqLim)
  [SysMotTqCmdScaCdnd] -> SF004B_AssiSumLim/17(SysMotTqCmdSca)
  ThermMotTqLim/1 -> SF004B_AssiSumLim/18(ThermMotTqLim)
  [ThermRednFac] -> SF004B_AssiSumLim/19(ThermRednFac)
  [TqLoaCmd] -> SF004B_AssiSumLim/20(TqLoaCmd)
  Ground3/1 -> SF004B_AssiSumLim/21(TqSteerMtgtnCmd)
  [VehSpd] -> SF004B_AssiSumLim/22(VehSpd)
  VehSpdMotTqLim/1 -> SF004B_AssiSumLim/23(VehSpdMotTqLim)
  Ground2/1 -> SF004B_AssiSumLim/24(WhlImbRejctnCmd)
  [GetNtcQlfrSts10] -> SF004B_AssiSumLim/25(GetNtcQlfrSts)
  [SetNtcSts10] -> SF004B_AssiSumLim/26(SetNtcSts)
  SF004B_AssiSumLim/3(MotTqCmdLimrMin) -> [MotTqCmdLimrMin]
  SF004B_AssiSumLim/4(MotTqCmdPreLim) -> [MotTqCmdPreLim]
  SF004B_AssiSumLim/5(SysProtnRednFac) -> [SysProtnRednFac]
  SF004B_AssiSumLim/6(SetManTqCmd) -> [SetManTqCmd]
  [FordMotTqCmdOvrl] -> SF004B_AssiSumLim/9(MotTqCmdOvrl)
  SF020B_PosnTrakgServo/1(PosnServoCmd) -> [PosnServoCmd]

== system Ford_T3T6_ArchCnctnDigrm/Generate Steering Command/Openloop Steering Command/System Protection ==
  note: ASIL B
  MotTqCmdLimdPreStall : Inport
  EoTProtection : Subsystem
  Motor Protection : Subsystem
  SF038A_LimrCdng : Subsystem  Tag=1.0.1  Description=This function provides a layer of protection from erroneous signals feeding into SF-04 Sum & Limit. It is applied primarily to limiting signals that serve to reduce motor torque command under certain operating conditions. This function can prevent step response or toggling behavior that might cause undesirable vehicle feel. It includes capability of fault injection at some inputs to facilitate tuning.
      settings: AttributesFormatString=Version: %<Tag>
  EotAssiSca : Outport
  EotActvCmd : Outport  Port=2
  EotDampgCmd : Outport  Port=3
  EotMotTqLim : Outport  Port=4
  StallMotTqLim : Outport  Port=5
  ThermMotTqLim : Outport  Port=6
  VehSpdMotTqLim : Outport  Port=7
  tag scope: SysMotTqCmdScaCdnd=global, ThermMotTqLimCdnd=global
  wires:
  EoTProtection/3(EotAssiSca) -> SF038A_LimrCdng/1(EotAssiSca)
  EoTProtection/4(EotMotTqLim) -> SF038A_LimrCdng/2(EotMotTqLim)
  Motor Protection/1(StallMotTqLim) -> SF038A_LimrCdng/3(StallMotTqLim)
  Motor Protection/2(ThermMotTqLim) -> SF038A_LimrCdng/5(ThermMotTqLim)
  SF038A_LimrCdng/1(EotAssiScaCdnd) -> EotAssiSca/1
  EoTProtection/1(EotActvCmd) -> EotActvCmd/1
  EoTProtection/2(EotDampgCmd) -> EotDampgCmd/1
  MotTqCmdLimdPreStall/1 -> Motor Protection/1(MotTqCmdLimdPreStall)
  [VehSpd] -> SF038A_LimrCdng/6(VehSpd)
  [FltInj_f32] -> SF038A_LimrCdng/8(FltInj_f32)
  SF038A_LimrCdng/2(EotMotTqLimCdnd) -> EotMotTqLim/1
  SF038A_LimrCdng/3(StallMotTqLimCdnd) -> StallMotTqLim/1
  SF038A_LimrCdng/5(ThermMotTqLimCdnd) -> [ThermMotTqLimCdnd], ThermMotTqLim/1
  SF038A_LimrCdng/6(VehSpdMotTqLimCdnd) -> VehSpdMotTqLim/1
  SF038A_LimrCdng/4(SysMotTqCmdScaCdnd) -> [SysMotTqCmdScaCdnd]
  EoTProtection/5(VehSpdMotTqLim) -> SF038A_LimrCdng/7(VehSpdMotTqLim)
  [SysMotTqCmdSca] -> SF038A_LimrCdng/4(SysMotTqCmdSca)

== system Ford_T3T6_ArchCnctnDigrm/Monitor System/Inferred Signals/HwAg before IMC ==
  note: Will be replaced by MotAgMeclIdptSig ES249A
  note: Used by GM
      | CF018
      |
      | Do we need it in Ford??
  note: May be from power limiter
  note: ASIL D
  note: ASIL D
  note: ASIL D
  note: RID 200F
  note: Do we have to use this as input for all SFs?
  note: CF075
  note: Not Required
  HwAgMeas : Inport
  HwAgIdptSig : Inport  Port=2
  HwTq : Inport  Port=3
  CF075A_FordHwAgArbn : Subsystem  Tag=1.1.0  Description=The purpose of Ford Handwheel Angle Arbitration is to use brakes data for position andcenter for Eletric Power Steering functionality.
      settings: AttributesFormatString=Version: %<Tag>
  SF041A_CmplncErr : Subsystem  Tag=1.1.0  Description=This function calculates the compliance error that can be used to compensate force and stiffness in the torque path between the motor position sensor and column axis.
      settings: AttributesFormatString=Version: %<Tag>
  SF042A_HwAgSnsrls : Subsystem  Tag=3.1.0  Description=This function determines whether the hand wheel should be autocentered using a low or high speed algorithm, or the last stored pinion angle. Once the correct algorithm is determined, it is used to center the handwheel.
      settings: AttributesFormatString=Version: %<Tag>
  SF045A_HwAgSysArbn : Subsystem  Tag=2.8.0  Description=This function accepts inputs from the various angle sources available in the EPS system and selects the angle source to be used for the system handwheel angle value. It also provides for compliance compensation of the angle value and determines the angle value and angle validity to be output on the vehicle data bus.
      settings: AttributesFormatString=Version: %<Tag>
  PinionAg : Outport
  PinionAgConf : Outport  Port=2
  tag scope: CmplncErrMotToPinion=global, CmplncErrPinionToHw=global, FSnsrlsHwCentr=global, FordCmpdHwPosn=global, FordCmpdHwPosnQlyFac=global, FordHwVel=global, FordHwVelVld=global, FordPosnOffsVld=global, FordRelHwPosn=global, FordRelHwPosnVld=global, HwAgAuthy=global, HwAgFinal=global, HwAgNotCorrd=global, HwAgSnsrls=global, HwAgSnsrlsConf=global, HwAgToSerlCom=global, HwAgVldToSerlCom=global, HwVel=global, HwVelToSerlCom=global, PinionAgArbn=global, PinionAgConf=global, PinionVel=global, PinionVelConf=global, RstSnsrlsHwCentr=global
  wires:
  SF045A_HwAgSysArbn/7(PinionAg) -> [PinionAgArbn], PinionAg/1
  SF045A_HwAgSysArbn/8(PinionAgConf) -> [PinionAgConf], [HwAgAuthy], PinionAgConf/1
  [CmplncErrMotToPinion] -> SF042A_HwAgSnsrls/1(CmplncErrMotToPinion)
  [HwTq] -> SF042A_HwAgSnsrls/2(HwTq)
  [MotAgCumvAlgndCrf] -> SF042A_HwAgSnsrls/3(MotAgCumvAlgndCrf)
  [MotAgCumvAlgndVld] -> SF042A_HwAgSnsrls/4(MotAgCumvAlgndVld)
  [MotAgMeclIdptSig] -> SF042A_HwAgSnsrls/5(MotAgMeclIdptSig)
  [MotTqCmdCrfDampd] -> SF042A_HwAgSnsrls/6(MotTqCmdCrf)
  [MotVelCrf] -> SF042A_HwAgSnsrls/7(MotVelCrf)
  [PinionAgArbn] -> SF042A_HwAgSnsrls/8(PinionAg)
  [PinionAgConf] -> SF042A_HwAgSnsrls/9(PinionAgConf)
  [VehSpd] -> SF042A_HwAgSnsrls/10(VehSpd)
  [VehSpdVld] -> SF042A_HwAgSnsrls/11(VehSpdVld)
  [VehYawRate] -> SF042A_HwAgSnsrls/12(VehYawRate)
  [VehYawRateVld] -> SF042A_HwAgSnsrls/13(VehYawRateVld)
  [WhlFrqVld] -> SF042A_HwAgSnsrls/14(WhlFrqVld)
  [WhlLeFrq] -> SF042A_HwAgSnsrls/15(WhlLeFrq)
  [WhlRiFrq] -> SF042A_HwAgSnsrls/16(WhlRiFrq)
  [GetNtcQlfrSts] -> SF042A_HwAgSnsrls/17(GetNtcQlfrSts)
  [GetRefTmr100MicroSec32bit] -> SF042A_HwAgSnsrls/18(GetRefTmr100MicroSec32bit)
  [GetTiSpan100MicroSec32bit] -> SF042A_HwAgSnsrls/19(GetTiSpan100MicroSec32bit)
  [StordLstPrm_SetRamBlockStatus] -> SF042A_HwAgSnsrls/20(StordLstPrm_SetRamBlockStatus)
  SF042A_HwAgSnsrls/1(HwAgSnsrls) -> [HwAgSnsrls]
  SF042A_HwAgSnsrls/2(HwAgSnsrlsConf) -> [HwAgSnsrlsConf]
  SF042A_HwAgSnsrls/3(FSnsrlsHwCentr) -> [FSnsrlsHwCentr]
  SF042A_HwAgSnsrls/4(RstSnsrlsHwCentr) -> [RstSnsrlsHwCentr]
  [HwTq] -> SF041A_CmplncErr/1(HwTq)
  [MotTqCmdPwrLimd] -> SF041A_CmplncErr/2(MotTqCmdCrf)
  SF041A_CmplncErr/1(CmplncErrMotToPinion) -> [CmplncErrMotToPinion]
  SF041A_CmplncErr/2(CmplncErrPinionToHw) -> [CmplncErrPinionToHw]
  [CmplncErrPinionToHw] -> SF045A_HwAgSysArbn/1(CmplncErrPinionToHw)
  HwAgMeas/1 -> SF045A_HwAgSysArbn/3(HwAgCorrd), SF045A_HwAgSysArbn/2(HwAg)
  [HwAgSnsrls] -> SF045A_HwAgSysArbn/5(HwAgSnsrls)
  [HwAgSnsrlsConf] -> SF045A_HwAgSysArbn/6(HwAgSnsrlsConf)
  HwTq/1 -> SF045A_HwAgSysArbn/7(HwTq)
  [MotVelCrf] -> SF045A_HwAgSysArbn/8(MotVelCrf)
  [MotVelVld] -> SF045A_HwAgSysArbn/9(MotVelVld)
  [GetNtcQlfrSts] -> SF045A_HwAgSysArbn/10(GetNtcQlfrSts)
  [FltInj_f32] -> SF045A_HwAgSysArbn/11(FltInj_f32)
  [GetRefTmr100MicroSec32bit] -> SF045A_HwAgSysArbn/12(GetRefTmr100MicroSec32bit)
  [GetTiSpan100MicroSec32bit] -> SF045A_HwAgSysArbn/13(GetTiSpan100MicroSec32bit)
  [SetNtcSts] -> SF045A_HwAgSysArbn/14(SetNtcSts)
  SF045A_HwAgSysArbn/1(HwAgFinal) -> [HwAgFinal]
  SF045A_HwAgSysArbn/2(HwAgNotCorrd) -> [HwAgNotCorrd]
  SF045A_HwAgSysArbn/3(HwAgToSerlCom) -> [HwAgToSerlCom]
  SF045A_HwAgSysArbn/4(HwAgVldToSerlCom) -> [HwAgVldToSerlCom]
  SF045A_HwAgSysArbn/5(HwVel) -> [HwVel]
  SF045A_HwAgSysArbn/6(HwVelToSerlCom) -> [HwVelToSerlCom]
  SF045A_HwAgSysArbn/9(PinionVel) -> [PinionVel]
  SF045A_HwAgSysArbn/10(PinionVelConf) -> [PinionVelConf]
  [FordAbsPrsnt] -> CF075A_FordHwAgArbn/9(FordAbsPrsnt)
  [PinionVel] -> CF075A_FordHwAgArbn/7(PinionVel)
  [FordVehSteerPinionAgOffs] -> CF075A_FordHwAgArbn/1(FordVehSteerPinionAgOffs)
  [FordVehSteerPinionOffsSts] -> CF075A_FordHwAgArbn/2(FordVehSteerPinionOffsSts)
  [FordVehSteerPinionOffsChks] -> CF075A_FordHwAgArbn/3(FordVehSteerPinionOffsChks)
  [FordVehSteerPinionOffsCnt] -> CF075A_FordHwAgArbn/4(FordVehSteerPinionOffsCnt)
  [FordSteerAgClrFlg] -> CF075A_FordHwAgArbn/10(FordSteerAgClrFlg)
  [HwAgNotCorrd] -> CF075A_FordHwAgArbn/6(HwAgNotCorrd)
  [GetRefTmr100MicroSec32bit] -> CF075A_FordHwAgArbn/12(GetRefTmr100MicroSec32bit)
  [GetTiSpan100MicroSec32bit] -> CF075A_FordHwAgArbn/13(GetTiSpan100MicroSec32bit)
  [NvMProxy_GetErrorStatus] -> CF075A_FordHwAgArbn/14(NonAbsOffsVldFlg_GetErrorStatus)
  [NvMProxy_SetRamBlockStatus] -> CF075A_FordHwAgArbn/15(NonAbsOffsVldFlg_SetRamBlockStatus)
  [NvMProxy_GetErrorStatus] -> CF075A_FordHwAgArbn/16(NonAbsOffs_GetErrorStatus)
  [NvMProxy_SetRamBlockStatus] -> CF075A_FordHwAgArbn/17(NonAbsOffs_SetRamBlockStatus)
  [NvMProxy_GetErrorStatus] -> CF075A_FordHwAgArbn/18(PrevIgnCycVal_GetErrorStatus)
  [NvMProxy_SetRamBlockStatus] -> CF075A_FordHwAgArbn/19(PrevIgnCycVal_SetRamBlockStatus)
  [SetNtcSts] -> CF075A_FordHwAgArbn/20(SetNtcSts)
  CF075A_FordHwAgArbn/1(FordCmpdHwPosn) -> [FordCmpdHwPosn]
  CF075A_FordHwAgArbn/2(FordCmpdHwPosnQlyFac) -> [FordCmpdHwPosnQlyFac]
  CF075A_FordHwAgArbn/4(FordHwVelVld) -> [FordHwVelVld]
  CF075A_FordHwAgArbn/5(FordPosnOffsVld) -> [FordPosnOffsVld]
  CF075A_FordHwAgArbn/6(FordRelHwPosn) -> [FordRelHwPosn]
  CF075A_FordHwAgArbn/7(FordRelHwPosnVld) -> [FordRelHwPosnVld]
  HwAgIdptSig/1 -> CF075A_FordHwAgArbn/11(HwAgIdptSig), SF045A_HwAgSysArbn/4(HwAgIdptSig)
  [PinionVelConf] -> CF075A_FordHwAgArbn/8(PinionVelConf)
  [HwAgFinal] -> CF075A_FordHwAgArbn/5(HwAgFinal)
  CF075A_FordHwAgArbn/3(FordHwVel) -> [FordHwVel]

== system Ford_T3T6_ArchCnctnDigrm/Monitor System/Inferred Signals/SF006A_TEstimn ==
  AmbT : Inport
  AmbTVld : Inport  Port=2
  AssiMechTEstimnDi : Inport  Port=3
  DualEcuFltMtgtnEna : Inport  Port=4
  EcuTFild : Inport  Port=5
  EngOilT : Inport  Port=6
  EngOilTVld : Inport  Port=7
  HwVel : Inport  Port=8
  IgnTiOff : Inport  Port=9
  MotAndThermProtnLoaMod : Inport  Port=10
  MotCurrPeakEstimd : Inport  Port=11
  VehTiVld : Inport  Port=12
  TFilStVal_GetErrorStatus : Inport  Port=13
  TFilStVal_SetRamBlockStatus : Inport  Port=14
  AssiMechT : Outport
  MotFetT : Outport  Port=2
  MotMagT : Outport  Port=3
  MotWidgT : Outport  Port=4

== system Ford_T3T6_ArchCnctnDigrm/Monitor System/Inferred Signals/SF007A_SysFricLrng ==
  AssiMechT : Inport
  FricLrngCustEna : Inport  Port=2
  FricLrngDi : Inport  Port=3
  HwAg : Inport  Port=4
  HwAgAuthy : Inport  Port=5
  HwTq : Inport  Port=6
  HwVel : Inport  Port=7
  MotTqCmdCrf : Inport  Port=8
  VehLatA : Inport  Port=9
  VehSpd : Inport  Port=10
  VehSpdVld : Inport  Port=11
  FltInj_f32 : Inport  Port=12
  FricLrngData_SetRamBlockStatus : Inport  Port=13
  FricNonLrngData_SetRamBlockStatus : Inport  Port=14
  GetNtcQlfrSts : Inport  Port=15
  GetRefTmr100MicroSec32bit : Inport  Port=16
  GetTiSpan100MicroSec32bit : Inport  Port=17
  SetNtcSts : Inport  Port=18
  MaxLrndFric : Outport
  SysFricEstimd : Outport  Port=2
  SysFricOffs : Outport  Port=3
  SysSatnFricEstimd : Outport  Port=4
  ClrFricLrngOperMod : Outport  Port=5
  FricLrngShtDwn : Outport  Port=6
  GetFricData : Outport  Port=7
  GetFricLrngData : Outport  Port=8
  GetFricOffsOutpDi : Outport  Port=9
  InitFricLrngTbl : Outport  Port=10
  SetFricData : Outport  Port=11
  SetFricLrngData : Outport  Port=12
  SetFricOffsOutpDi : Outport  Port=13

== system Ford_T3T6_ArchCnctnDigrm/Monitor System/Inferred Signals/SF011A_EotLrng ==
  HwAg : Inport
  HwAgAuthy : Inport  Port=2
  HwAgDiDiagSts : Inport  Port=3
  HwAgEotSig0Avl : Inport  Port=4
  HwAgEotSig0Ccw : Inport  Port=5
  HwAgEotSig0Cw : Inport  Port=6
  HwAgEotSig1Avl : Inport  Port=7
  HwAgEotSig1Ccw : Inport  Port=8
  HwAgEotSig1Cw : Inport  Port=9
  HwTq : Inport  Port=10
  MotVelCrf : Inport  Port=11
  EotNvmData_GetErrorStatus : Inport  Port=12
  EotNvmData_SetRamBlockStatus : Inport  Port=13
  GetNtcQlfrSts : Inport  Port=14
  GetRefTmr100MicroSec32bit : Inport  Port=15
  GetTiSpan100MicroSec32bit : Inport  Port=16
  MaxHwAgCwAndCcw_GetErrorStatus : Inport  Port=17
  MaxHwAgCwAndCcw_SetRamBlockStatus : Inport  Port=18
  SetNtcSts : Inport  Port=19
  HwAgCcwDetd : Outport
  HwAgCwDetd : Outport  Port=2
  HwAgEotCcw : Outport  Port=3
  HwAgEotCw : Outport  Port=4
  GetHwAgOverTrvlCnt : Outport  Port=5
  RstHwAgOverTrvlCnt : Outport  Port=6
  RstMaxHwAgCwAndCcw : Outport  Port=7
  RtnMaxHwAgCwAndCcw : Outport  Port=8
  SerlComRstEot : Outport  Port=9
  SetHwAgOverTrvlCnt : Outport  Port=10

== system Ford_T3T6_ArchCnctnDigrm/Monitor System/Inferred Signals/SF040A_MotVel ==
  AssiMechPolarity : Inport
  MotAgBuf : Inport  Port=2
  MotAgBufIdx : Inport  Port=3
  MotAgMeclIdptSig : Inport  Port=4
  MotAgTiBuf : Inport  Port=5
  MotCtrlMotAgBuf_SigIn : Inport  Port=6
  MotCtrlMotAgMeasTi : Inport  Port=7
  MotCtrlMotAgMecl : Inport  Port=8
  MotCtrlMotAgTiBuf_SigIn : Inport  Port=9
  MotVelCrf : Outport
  MotVelMrf : Outport  Port=2
  MotVelVld : Outport  Port=3
  MotCtrlMotAgBufIdx : Outport  Port=4
  MotCtrlMotAgBuf_SigOut : Outport  Port=5
  MotCtrlMotAgTiBuf_SigOut : Outport  Port=6

== system Ford_T3T6_ArchCnctnDigrm/Monitor System/Inferred Signals/SF056A_DrvrTqEstimn ==
  AssiMechPolarity : Inport
  HwAg : Inport  Port=2
  HwTq : Inport  Port=3
  MotTqCmdPwrLimd : Inport  Port=4
  MotVelCrf : Inport  Port=5
  DrvrTqEstimd : Outport

== system Ford_T3T6_ArchCnctnDigrm/Monitor System/Inferred Signals/SF108A_MotCurrPeakEstimn ==
  DualEcuMotCtrlMtgtnEna : Inport
  MotAndThermProtnLoaMod : Inport  Port=2
  MotCurrDax : Inport  Port=3
  MotCurrDaxCmd : Inport  Port=4
  MotCurrQax : Inport  Port=5
  MotCurrQaxCmd : Inport  Port=6
  MotCurrPeakEstimd : Outport
  MotCurrPeakEstimdFild : Outport  Port=2

== system Ford_T3T6_ArchCnctnDigrm/Monitor System/Inferred Signals/SF109A_ElecPwrCns ==
  BrdgVltg : Inport
  MotAndThermProtnLoaMod : Inport  Port=2
  MotCurrDax : Inport  Port=3
  MotCurrDaxCmd : Inport  Port=4
  MotCurrQax : Inport  Port=5
  MotCurrQaxCmd : Inport  Port=6
  MotVltgDax : Inport  Port=7
  MotVltgQax : Inport  Port=8
  ElecInpPwrEstim : Outport
  SplyCurrEstim : Outport  Port=2
